simulink model "TwoLinkRobot"  (R2018b)
settings: Solver=VariableStepAuto  StartTime=0.0  StopTime=10.0  RelTol=1e-3
values from neighbouring files (symbols this model uses):
  alpha = 1    [tvnormaff.m]    (also in twoLinkInverseKinematics.m = RobotParam.alpha; twoLinkRobot_BuildLTVModel.m = 0.4425; twoLinkRobot_BuildLTVModel.mat = 0.4425)
  beta = sqrt((alpha^2-alphaMaxSq)/lambda1)    [tvnormaff.m]    (also in twoLinkInverseKinematics.m = RobotParam.beta; twoLinkRobot_BuildLTVModel.m = 0.09; twoLinkRobot_BuildLTVModel.mat = 0.09)
  delta = RobotParam.delta    [twoLinkInverseKinematics.m]    (also in twoLinkRobot_BuildLTVModel.m = 0.105; twoLinkRobot_BuildLTVModel.mat = 0.105)
  eta0 = tvsubs(etabar,T0)    [twoLinkRobot_BuildLTVModel.m]    (also in twoLinkRobot_BuildLTVModel.mat = [-2.4644416189 -1.15647760714 -0.00295563019952 0.0032893506)
settings Model: Creator=jyotbuch  LastModifiedBy=jyotbuch
settings ModelReferenceCC: ModelReferenceMinAlgLoopOccurrences=on

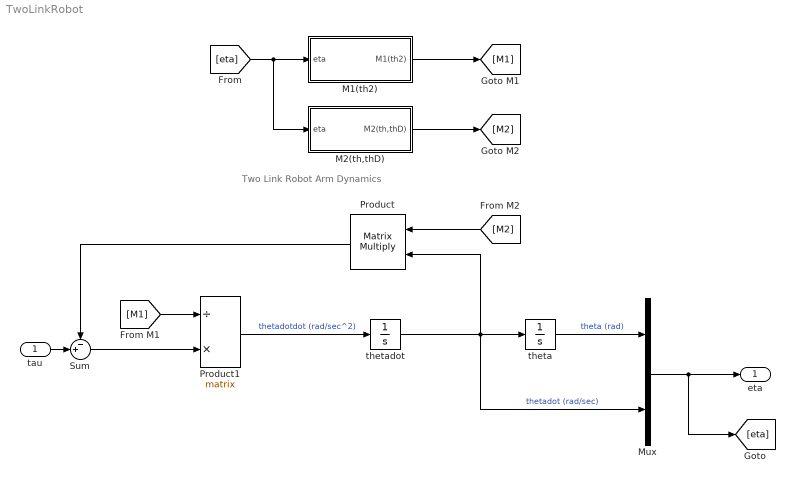
== system TwoLinkRobot ==
  note: Two Link Robot Arm Dynamics
  tau : Inport  PortDimensions=2
  M1(th2) : Subsystem  TreatAsAtomicUnit=on
  M2(th,thD) : Subsystem  TreatAsAtomicUnit=on
  Mux : Mux  Inputs=2
  Product : Product  Inputs=**  Multiplication=Matrix(*)
  Product1 : Product  Inputs=/*  Multiplication=Matrix(*)
  Sum : Sum  Inputs=-+|
  theta : Integrator  InitialCondition=eta0(1:2)
  thetadot : Integrator  InitialCondition=eta0(3:4)
  eta : Outport
  wires:
  tau/1 -> Sum/2
  theta/1 -> Mux/1  "theta (rad)"
  Mux/1 -> [eta], eta/1
  M2(th,thD)/1(M2(th,thD)) -> [M2]
  [eta] -> M2(th,thD)/1(eta), M1(th2)/1(eta)
  M1(th2)/1(M1(th2)) -> [M1]
  [M2] -> Product/1
  Product/1 -> Sum/1
  Sum/1 -> Product1/2
  [M1] -> Product1/1
  thetadot/1 -> Mux/2, Product/2, theta/1  "thetadot (rad/sec)"
  Product1/1 -> thetadot/1  "thetadotdot (rad/sec^2)"

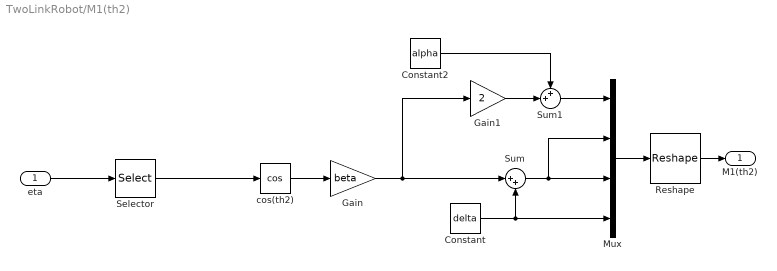
== system TwoLinkRobot/M1(th2) ==
  eta : Inport
  Constant : Constant  Value=delta
  Constant2 : Constant  Value=alpha
  Gain : Gain  Gain=beta
  Gain1 : Gain  Gain=2
  Mux : Mux
  Reshape : Reshape  OutputDimensionality=Customize  OutputDimensions=[2 2]
  Selector : Selector  InputPortWidth=4  IndexOptions=Index vector (dialog)  Indices=2  OutputSizes=1
  Sum : Sum  Inputs=|++
  Sum1 : Sum  Inputs=++|
  cos(th2) : Trigonometry  Operator=cos
  M1(th2) : Outport
  wires:
  Reshape/1 -> M1(th2)/1
  Mux/1 -> Reshape/1
  Constant/1 -> Mux/4, Sum/2
  Sum/1 -> Mux/3, Mux/2
  cos(th2)/1 -> Gain/1
  Gain/1 -> Gain1/1, Sum/1
  Constant2/1 -> Sum1/1
  Sum1/1 -> Mux/1
  Gain1/1 -> Sum1/2
  eta/1 -> Selector/1
  Selector/1 -> cos(th2)/1

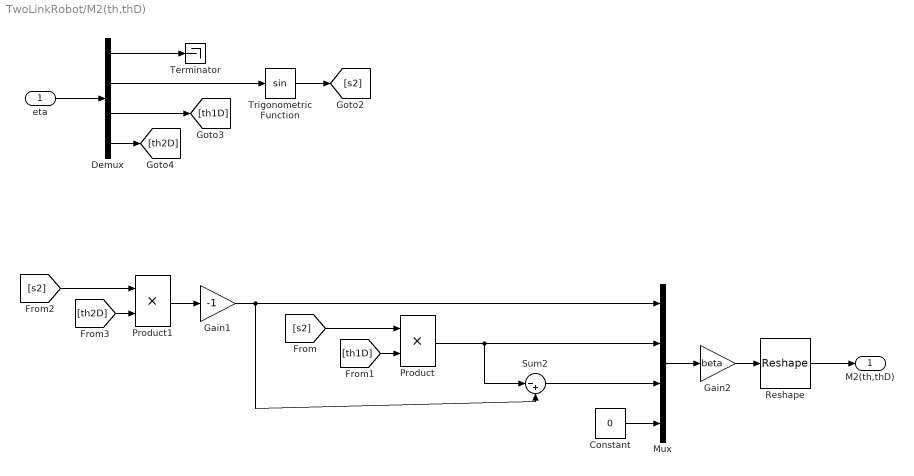
== system TwoLinkRobot/M2(th,thD) ==
  eta : Inport
  Constant : Constant  Value=0
  Demux : Demux
  Gain1 : Gain  Gain=-1
  Gain2 : Gain  Gain=beta
  Mux : Mux
  Product : Product
  Product1 : Product
  Reshape : Reshape  OutputDimensionality=Customize  OutputDimensions=[2 2]
  Sum2 : Sum  Inputs=|-+
  Terminator : Terminator
  Trigonometric Function : Trigonometry
  M2(th,thD) : Outport
  wires:
  Constant/1 -> Mux/4
  Reshape/1 -> M2(th,thD)/1
  eta/1 -> Demux/1
  Demux/4 -> [th2D]
  Demux/1 -> Terminator/1
  Demux/2 -> Trigonometric Function/1
  Demux/3 -> [th1D]
  Trigonometric Function/1 -> [s2]
  [s2] -> Product/1
  [th1D] -> Product/2
  Product/1 -> Sum2/1, Mux/2
  Gain2/1 -> Reshape/1
  Mux/1 -> Gain2/1
  [th2D] -> Product1/2
  [s2] -> Product1/1
  Product1/1 -> Gain1/1
  Sum2/1 -> Mux/3
  Gain1/1 -> Sum2/2, Mux/1
